simulink model "cruise_control"  (R2013a)
settings: Solver=ode45  StartTime=0.0  StopTime=10.0  RelTol=1e-3
PreLoadFcn:
  | load('cruise_control.mat')
values from neighbouring files (symbols this model uses):
  Ki = 1    [cruise_control.mat]
  Kp = 1    [cruise_control.mat]
settings Model: Creator=luca  LastModifiedBy=luca

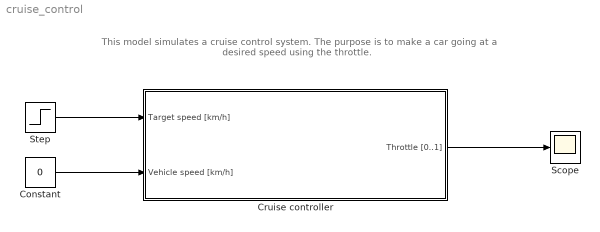
== system cruise_control ==
  note: This model simulates a cruise control system.
      | The purpose is to make a car going at a desired
      | speed using the throttle.
  Constant : Constant  Value=0
  Cruise controller : Subsystem
  Scope : Scope
  Step : Step  After=0.1  SampleTime=0
  wires:
  Cruise controller/1(Throttle [0..1]) -> Scope/1
  Step/1 -> Cruise controller/1(Target speed [km/h])
  Constant/1 -> Cruise controller/2(Vehicle speed [km/h])

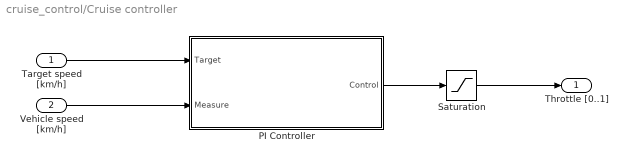
== system cruise_control/Cruise controller ==
  Target speed [km/h] : Inport
  Vehicle speed [km/h] : Inport  Port=2
  PI Controller : Subsystem
  Saturation : Saturate  UpperLimit=1  LowerLimit=0
  Throttle [0..1] : Outport
  wires:
  Vehicle speed [km/h]/1 -> PI Controller/2(Measure)
  PI Controller/1(Control) -> Saturation/1
  Saturation/1 -> Throttle [0..1]/1
  Target speed [km/h]/1 -> PI Controller/1(Target)

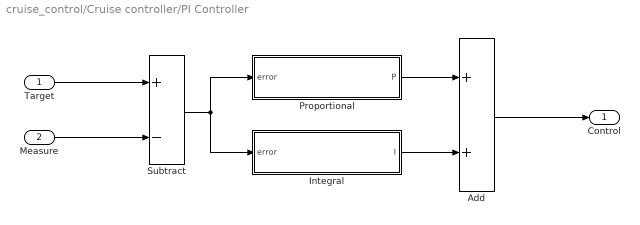
== system cruise_control/Cruise controller/PI Controller ==
  Target : Inport
  Measure : Inport  Port=2
  Add : Sum
  Integral : Subsystem
  Proportional : Subsystem
  Subtract : Sum  Inputs=+-
  Control : Outport
  wires:
  Subtract/1 -> Integral/1(error), Proportional/1(error)
  Target/1 -> Subtract/1
  Measure/1 -> Subtract/2
  Integral/1(I) -> Add/2
  Proportional/1(P) -> Add/1
  Add/1 -> Control/1

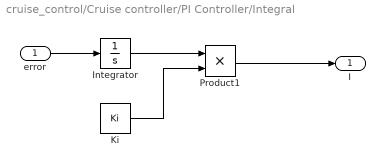
== system cruise_control/Cruise controller/PI Controller/Integral ==
  error : Inport
  Integrator : Integrator
  Ki : Constant  Value=Ki
  Product1 : Product
  I : Outport
  wires:
  Ki/1 -> Product1/2
  Integrator/1 -> Product1/1
  Product1/1 -> I/1
  error/1 -> Integrator/1

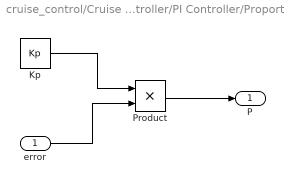
== system cruise_control/Cruise controller/PI Controller/Proportional ==
  error : Inport
  Kp : Constant  Value=Kp
  Product : Product
  P : Outport
  wires:
  Kp/1 -> Product/1
  Product/1 -> P/1
  error/1 -> Product/2
